simulink model "white_box"  (R2024b)
settings: Solver=ode1  StartTime=0.0  StopTime=Tobs  FixedStep=Ts  RelTol=1e-3
values from neighbouring files (symbols this model uses):
  delta_t = 10E-6    (= 1e-05)    [main_SVD.m]    (also in main_scan_FD.m)
  f0 = 50    [main_SVD.m]    (also in main_scan_FD.m)
  Id_ss = 0    [main_scan_FD.m]
  Ipeak = Sbase/Vpeak    [main_scan_FD.m]
  Iq_ss = 0    [main_scan_FD.m]
  P_finalvalue = 0.486    [main_scan_FD.m]    (also in main_ss_composite.m = 0.05)
  P_step_time = 1.5    [main_scan_FD.m]    (also in main_ss_composite.m = 10)
  phi = 0 * pi / 180    (= 0)    [main_SVD.m]
  signal_type = 1    [main_scan_FD.m]
  Ts = delta_t    (= 1e-05)    [main_scan_FD.m]
  V_finalvalue = 0.99    [main_ss_composite.m]
  V_step_time = 100    [main_scan_FD.m]    (also in main_ss_composite.m = 10)
  Vd_ss = 0    [main_scan_FD.m]
  Vpeak = (Vbase/sqrt(3))*sqrt(2)    [main_scan_FD.m]
  Vq_ss = 0    [main_scan_FD.m]
undefined symbols (not defined in the file or in its folder): C_dc, C_filt, dist_time, dist_value_0, dist_value_a, dist_value_b, dist_value_c, dist_value_d, dist_value_n, dist_value_p, dist_value_q, fd, I_charge, Iss_type, ki_inner_d_pu, ki_inner_q_pu, ki_outer_P_pu, ki_outer_V_pu, ki_pll, kp_inner_d_pu, kp_inner_q_pu, kp_outer_P_pu, kp_outer_V_pu, kp_pll, L, L_base, L_grid, L_vsc, omega_b, P_base, R_grid, R_vsc, Rsource, t_charge, V_base, V_dc, Vss_type
libraries: spsThreePhaseVIMeasurementLib x19, spsControlledVoltageSourceLib x18, spsControlledCurrentSourceLib x14, slpidlib x5, spsThreePhaseSeriesRLCBranchLib x5, spsabctodq0Lib x4, spsGroundLib x3, eeGeneralControl x2, spsdq0toabcLib x2, simulink x2, spsLeadLagFilterLib x1, spsParallelRLCBranchLib x1
(part 1 of 3)
settings Model: SimulationMode=accelerator  Creator=osro  LastModifiedBy=nicolae.darii
settings SolverCC: AlgebraicLoopSolver=TrustRegion
settings DebuggingCC: UnconnectedInputMsg=warning  UnconnectedOutputMsg=warning  UnconnectedLineMsg=warning
settings ModelReferenceCC: EnableRefExpFcnMdlSchedulingChecks=on
settings RTWCC: GPUComputeCapability=3.5

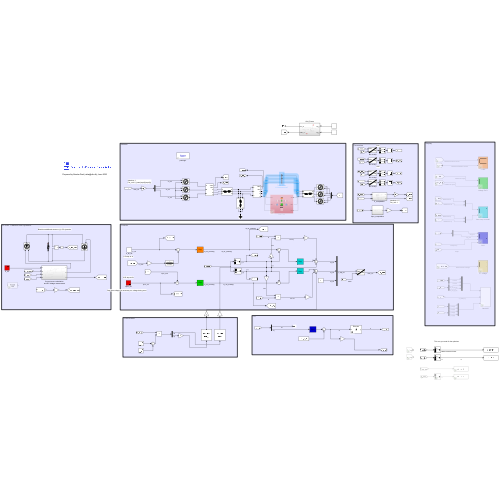
[thumbnail: Simulink's stored preview of the top-level diagram]
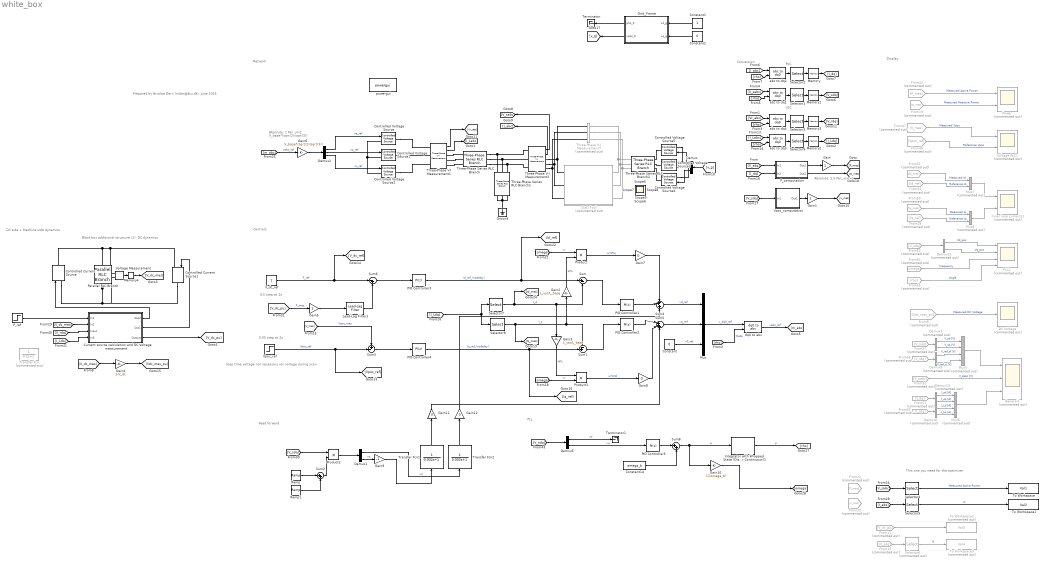
== system white_box ==
  note: Feed forward
  note: Step time voltage not necessary vor voltage during scan
  note: This one you need for the optimizer
  note: PLL
  note: 0.05 step at 2s
  note: 0.5 step at 1s
  note: Absolute: 1.5
      | Per_unit: 1
  note: Absolute: 1
      | Per_unit: V_base*(sqrt(2)/sqrt(3))
  note: Conversion
  note: Controls
  note: Network
  note: VSC
  note: PoC
  note: Prepared by Nicolae Darii (nidar@dtu.dk), June 2025
  note: DC side + Machine side dynamics
  note: Black box additional structure (1): DC dynamics
  note: Display
  Constant : Constant  Value=0
  Constant1 : Constant
  Constant14 : Constant  Value=omega_b
  Constant2 : Constant  Value=0
  Controlled Current Source : spsControlledCurrentSourceLib/Controlled Current Source  Initialize=on  Source_Type=AC  Amplitude=0  Phase=0  Frequency=0  Measurements=None
  Controlled Current Source1 : spsControlledCurrentSourceLib/Controlled Current Source  Initialize=on  Source_Type=AC  Amplitude=0  Phase=0  Frequency=0  Measurements=None
  Controlled Voltage Source{,1..5} (6 alike) : spsControlledVoltageSourceLib/Controlled Voltage Source  Initialize=on  Source_Type=AC  Amplitude=0  Phase=0  Frequency=0  Measurements=None
  Current source calculation and DC Voltage measurement : Subsystem
  DC Voltage : Scope  Commented=on
  Demux : Demux  Outputs=3
  Demux1 : Demux  Outputs=2
  Demux{7..11} (5 alike) : Demux  Commented=on  Outputs=2
  Demux2 : Demux  Outputs=3
  Demux5 : Demux  Outputs=2
  From11 : From  Commented=on  GotoTag=V_dc_pu
  From12 : From  Commented=on  GotoTag=V_sdq
  From19 : From  Commented=on  GotoTag=Q_mes
  From20 : From  Commented=on  GotoTag=V_mes
  From22 : From  Commented=on  GotoTag=P_mes
  From32 : From  Commented=on  GotoTag=V_sabc
  From35 : From  Commented=on  GotoTag=I_Ldq
  From37 : From  Commented=on  GotoTag=V_sdq
  From42 : From  Commented=on  GotoTag=P_mes
  From47 : From  Commented=on  GotoTag=V_mes
  From48 : From  Commented=on  GotoTag=Vpoc_ref
  From49 : From  Commented=on  GotoTag=Iq_ref
  From50 : From  Commented=on  GotoTag=Iq_mes
  From51 : From  Commented=on  GotoTag=Id_mes
  From52 : From  Commented=on  GotoTag=Id_ref
  From53 : From  Commented=on  GotoTag=V_sdq
  From54 : From  Commented=on  GotoTag=omega
  From55 : From  Commented=on  GotoTag=rho
  From56 : From  Commented=on  GotoTag=V_rdq
  From57 : From  Commented=on  GotoTag=I_dq
  From9 : From  Commented=on  GotoTag=Vdc_mes_pu
  Gain : Gain
  Gain1 : Gain
  Gain10 : Gain  Gain=1/(omega_b)
  Gain{7..8,11..12} (4 alike) : Gain  Gain=0
  Gain2 : Gain  Gain=L_vsc/L_base
  Gain3 : Gain  Gain=L_vsc/L_base
  Gain4 : Gain  Gain=1/V_dc
  Gain5 : Gain
  Gain6 : Gain  Gain=V_base*(sqrt(2)/sqrt(3))
  Gain9 : Gain  Gain=-1
  General1 : Scope  Commented=on  NumInputPorts=3
  Grid_Frame : Subsystem
  Ground : spsGroundLib/Ground  LConnTagsString=a
  Inner loop currents1 : Scope  Commented=on  NumInputPorts=2
  Integrator with Wrapped State (Discrete or Continuous)1 : eeGeneralControl/Integrator with Wrapped State (Discrete or Continuous)  LabelModeActiveChoice=Discrete  WrappedStateUpperValue=2*pi  WrappedStateLowerValue=0  x0=0  Ts=-1
  Lead-Lag Filter1 : spsLeadLagFilterLib/Lead-Lag Filter  T1=T1  T2=T2  Vdc_Init=1  Ts=Ts
      settings: LibrarySourceBlock=|
      | sps_lib/Control/Filters/Lead-Lag
      | Filter
  Memory{,1..3} (4 alike) : Memory  InitialCondition=[0 0]  InheritSampleTime=on  LinearizeMemory=on  LinearizeAsDelay=on
  Memory4 : Memory
  Mux : Mux  Inputs=3
  Mux5 : Mux  Commented=on
  Mux6 : Mux  Commented=on
  Mux7 : Mux  Commented=on  Inputs=2
  Mux8 : Mux  Commented=on  Inputs=2
  PID Controller1 : slpidlib/PID Controller  Controller=PI  Form=Parallel  TimeDomain=Discrete-time  UseExternalTs=off  SampleTime=Ts  IntegratorMethod=Forward Euler  FilterMethod=Forward Euler  ControllerParametersSource=internal  P=kp_inner_d_pu  I=ki_inner_d_pu  UseKiTs=off  D=0  UseExternalDerivativeSource=off  N=100  UseFilter=on  TunerSelectOption=Transfer Function Based (PID Tuner App)  InitialConditionSource=internal  InitialConditionForIntegrator=0  InitialConditionForFilter=0  DifferentiatorICPrevScaledInput=0  ExternalReset=none  TrackingMode=off  Kt=1  LimitOutput=off  SatLimitsSource=internal  UpperSaturationLimit=inf  LowerSaturationLimit=-inf  LinearizeAsGain=on  AntiWindupMode=none  Kb=1  LimitIntegrator=off  UpperIntegratorSaturationLimit=inf  LowerIntegratorSaturationLimit=-inf  POutMin=[]  POutMax=[]  IOutMin=[]  IOutMax=[]  DOutMin=[]  DOutMax=[]  NOutMin=[]  NOutMax=[]  SumOutMin=[]  SumOutMax=[]  SaturationOutMin=[]  SaturationOutMax=[]  PParamMin=[]  PParamMax=[]  IParamMin=[]  IParamMax=[]  DParamMin=[]  DParamMax=[]  NParamMin=[]  NParamMax=[]  KbParamMin=[]  KbParamMax=[]  KtParamMin=[]  KtParamMax=[]  KbOutMin=[]  KbOutMax=[]  KtOutMin=[]  KtOutMax=[]  IntegratorOutMin=[]  IntegratorOutMax=[]  FilterOutMin=[]  FilterOutMax=[]  SumI1OutMin=[]  SumI1OutMax=[]  SumI2OutMin=[]  SumI2OutMax=[]  SumI3OutMin=[]  SumI3OutMax=[]  SumI4OutMin=[]  SumI4OutMax=[]  SumDOutMin=[]  SumDOutMax=[]  DifferentiatorOutMin=[]  DifferentiatorOutMax=[]  FilterDiffOutCoefMin=[]  FilterDiffOutCoefMax=[]  ReciprocalOutMin=[]  ReciprocalOutMax=[]  SumDenOutMin=[]  SumDenOutMax=[]  SumNumOutMin=[]  SumNumOutMax=[]  DivideOutMin=[]  DivideOutMax=[]  UdiffTsProdOutMin=[]  UdiffTsProdOutMax=[]  NTsProdOutMin=[]  NTsProdOutMax=[]  UintegralTsProdOutMin=[]  UintegralTsProdOutMax=[]  UngainTsProdOutMin=[]  UngainTsProdOutMax=[]  ClampingZeroOutDataTypeStr=Inherit: Inherit via back propagation  ClampingZeroOutMin=[]  ClampingZeroOutMax=[]  FilterDenConstantOutDataTypeStr=Inherit: Inherit via back propagation  FilterDenConstantOutMin=[]  FilterDenConstantOutMax=[]  PCopyOutDataTypeStr=Inherit: Inherit via back propagation  PCopyOutMin=[]  PCopyOutMax=[]  NCopyOutDataTypeStr=Inherit: Inherit via back propagation  NCopyOutMin=[]  NCopyOutMax=[]  IntegratorContinuousStateAttributes=''  IntegratorStateMustResolveToSignalObject=off  IntegratorRTWStateStorageClass=Auto  FilterContinuousStateAttributes=''  FilterStateMustResolveToSignalObject=off  FilterRTWStateStorageClass=Auto  ParallelPVariant=InternalParameters  IdealPVariant=Disabled  IVariant=InternalParameters  DVariant=Disabled  IntegratorVariant=Discrete  SatVariant=Disabled  AWVariant=Passthrough  PCopyVariant=Disabled  TRVariant=Disabled  FdbkBlocksVariant=Forward  IdealPFdbkVariant=Disabled  SatFdbkVariant=Disabled  DerivativeFilterVariant=Disabled  NVariant=Disabled  NCopyVariant=Disabled_SignalSpec  FilterICVariant=Disabled  IntegratorICVariant=InternalICs  ExternalResetVariant=Disabled  TRSumVariant=Passthrough  SumFdbkVariant=Disabled  SumVariant=Sum_PI  TsampFilterVariant=InternalTs  TsampNgainVariant=Passthrough  TsampIntegralVariant=Disabled_SignalSpec  ExternalSaturationOutDataTypeStr=Inherit: Same as second input  DerivativeSourceVariant=Disabled  PreIntVariant=InternalPreInt
  PID Controller2 : slpidlib/PID Controller  Controller=PI  Form=Parallel  TimeDomain=Discrete-time  UseExternalTs=off  SampleTime=Ts  IntegratorMethod=Forward Euler  FilterMethod=Forward Euler  ControllerParametersSource=internal  P=kp_inner_q_pu  I=ki_inner_q_pu  UseKiTs=off  D=0  UseExternalDerivativeSource=off  N=100  UseFilter=on  TunerSelectOption=Transfer Function Based (PID Tuner App)  InitialConditionSource=internal  InitialConditionForIntegrator=0  InitialConditionForFilter=0  DifferentiatorICPrevScaledInput=0  ExternalReset=none  TrackingMode=off  Kt=1  LimitOutput=off  SatLimitsSource=internal  UpperSaturationLimit=inf  LowerSaturationLimit=-inf  LinearizeAsGain=on  AntiWindupMode=none  Kb=1  LimitIntegrator=off  UpperIntegratorSaturationLimit=inf  LowerIntegratorSaturationLimit=-inf  POutMin=[]  POutMax=[]  IOutMin=[]  IOutMax=[]  DOutMin=[]  DOutMax=[]  NOutMin=[]  NOutMax=[]  SumOutMin=[]  SumOutMax=[]  SaturationOutMin=[]  SaturationOutMax=[]  PParamMin=[]  PParamMax=[]  IParamMin=[]  IParamMax=[]  DParamMin=[]  DParamMax=[]  NParamMin=[]  NParamMax=[]  KbParamMin=[]  KbParamMax=[]  KtParamMin=[]  KtParamMax=[]  KbOutMin=[]  KbOutMax=[]  KtOutMin=[]  KtOutMax=[]  IntegratorOutMin=[]  IntegratorOutMax=[]  FilterOutMin=[]  FilterOutMax=[]  SumI1OutMin=[]  SumI1OutMax=[]  SumI2OutMin=[]  SumI2OutMax=[]  SumI3OutMin=[]  SumI3OutMax=[]  SumI4OutMin=[]  SumI4OutMax=[]  SumDOutMin=[]  SumDOutMax=[]  DifferentiatorOutMin=[]  DifferentiatorOutMax=[]  FilterDiffOutCoefMin=[]  FilterDiffOutCoefMax=[]  ReciprocalOutMin=[]  ReciprocalOutMax=[]  SumDenOutMin=[]  SumDenOutMax=[]  SumNumOutMin=[]  SumNumOutMax=[]  DivideOutMin=[]  DivideOutMax=[]  UdiffTsProdOutMin=[]  UdiffTsProdOutMax=[]  NTsProdOutMin=[]  NTsProdOutMax=[]  UintegralTsProdOutMin=[]  UintegralTsProdOutMax=[]  UngainTsProdOutMin=[]  UngainTsProdOutMax=[]  ClampingZeroOutDataTypeStr=Inherit: Inherit via back propagation  ClampingZeroOutMin=[]  ClampingZeroOutMax=[]  FilterDenConstantOutDataTypeStr=Inherit: Inherit via back propagation  FilterDenConstantOutMin=[]  FilterDenConstantOutMax=[]  PCopyOutDataTypeStr=Inherit: Inherit via back propagation  PCopyOutMin=[]  PCopyOutMax=[]  NCopyOutDataTypeStr=Inherit: Inherit via back propagation  NCopyOutMin=[]  NCopyOutMax=[]  IntegratorContinuousStateAttributes=''  IntegratorStateMustResolveToSignalObject=off  IntegratorRTWStateStorageClass=Auto  FilterContinuousStateAttributes=''  FilterStateMustResolveToSignalObject=off  FilterRTWStateStorageClass=Auto  ParallelPVariant=InternalParameters  IdealPVariant=Disabled  IVariant=InternalParameters  DVariant=Disabled  IntegratorVariant=Discrete  SatVariant=Disabled  AWVariant=Passthrough  PCopyVariant=Disabled  TRVariant=Disabled  FdbkBlocksVariant=Forward  IdealPFdbkVariant=Disabled  SatFdbkVariant=Disabled  DerivativeFilterVariant=Disabled  NVariant=Disabled  NCopyVariant=Disabled_SignalSpec  FilterICVariant=Disabled  IntegratorICVariant=InternalICs  ExternalResetVariant=Disabled  TRSumVariant=Passthrough  SumFdbkVariant=Disabled  SumVariant=Sum_PI  TsampFilterVariant=InternalTs  TsampNgainVariant=Passthrough  TsampIntegralVariant=Disabled_SignalSpec  ExternalSaturationOutDataTypeStr=Inherit: Same as second input  DerivativeSourceVariant=Disabled  PreIntVariant=InternalPreInt
  PID Controller3 : slpidlib/PID Controller  Controller=PI  Form=Parallel  TimeDomain=Discrete-time  UseExternalTs=off  SampleTime=Ts  IntegratorMethod=Forward Euler  FilterMethod=Forward Euler  ControllerParametersSource=internal  P=kp_outer_P_pu  I=ki_outer_P_pu  UseKiTs=off  D=0  UseExternalDerivativeSource=off  N=100  UseFilter=on  TunerSelectOption=Transfer Function Based (PID Tuner App)  InitialConditionSource=internal  InitialConditionForIntegrator=0  InitialConditionForFilter=0  DifferentiatorICPrevScaledInput=0  ExternalReset=none  TrackingMode=off  Kt=1  LimitOutput=off  SatLimitsSource=internal  UpperSaturationLimit=inf  LowerSaturationLimit=-inf  LinearizeAsGain=on  AntiWindupMode=none  Kb=1  LimitIntegrator=off  UpperIntegratorSaturationLimit=inf  LowerIntegratorSaturationLimit=-inf  POutMin=[]  POutMax=[]  IOutMin=[]  IOutMax=[]  DOutMin=[]  DOutMax=[]  NOutMin=[]  NOutMax=[]  SumOutMin=[]  SumOutMax=[]  SaturationOutMin=[]  SaturationOutMax=[]  PParamMin=[]  PParamMax=[]  IParamMin=[]  IParamMax=[]  DParamMin=[]  DParamMax=[]  NParamMin=[]  NParamMax=[]  KbParamMin=[]  KbParamMax=[]  KtParamMin=[]  KtParamMax=[]  KbOutMin=[]  KbOutMax=[]  KtOutMin=[]  KtOutMax=[]  IntegratorOutMin=[]  IntegratorOutMax=[]  FilterOutMin=[]  FilterOutMax=[]  SumI1OutMin=[]  SumI1OutMax=[]  SumI2OutMin=[]  SumI2OutMax=[]  SumI3OutMin=[]  SumI3OutMax=[]  SumI4OutMin=[]  SumI4OutMax=[]  SumDOutMin=[]  SumDOutMax=[]  DifferentiatorOutMin=[]  DifferentiatorOutMax=[]  FilterDiffOutCoefMin=[]  FilterDiffOutCoefMax=[]  ReciprocalOutMin=[]  ReciprocalOutMax=[]  SumDenOutMin=[]  SumDenOutMax=[]  SumNumOutMin=[]  SumNumOutMax=[]  DivideOutMin=[]  DivideOutMax=[]  UdiffTsProdOutMin=[]  UdiffTsProdOutMax=[]  NTsProdOutMin=[]  NTsProdOutMax=[]  UintegralTsProdOutMin=[]  UintegralTsProdOutMax=[]  UngainTsProdOutMin=[]  UngainTsProdOutMax=[]  ClampingZeroOutDataTypeStr=Inherit: Inherit via back propagation  ClampingZeroOutMin=[]  ClampingZeroOutMax=[]  FilterDenConstantOutDataTypeStr=Inherit: Inherit via back propagation  FilterDenConstantOutMin=[]  FilterDenConstantOutMax=[]  PCopyOutDataTypeStr=Inherit: Inherit via back propagation  PCopyOutMin=[]  PCopyOutMax=[]  NCopyOutDataTypeStr=Inherit: Inherit via back propagation  NCopyOutMin=[]  NCopyOutMax=[]  IntegratorContinuousStateAttributes=''  IntegratorStateMustResolveToSignalObject=off  IntegratorRTWStateStorageClass=Auto  FilterContinuousStateAttributes=''  FilterStateMustResolveToSignalObject=off  FilterRTWStateStorageClass=Auto  ParallelPVariant=InternalParameters  IdealPVariant=Disabled  IVariant=InternalParameters  DVariant=Disabled  IntegratorVariant=Discrete  SatVariant=Disabled  AWVariant=Passthrough  PCopyVariant=Disabled  TRVariant=Disabled  FdbkBlocksVariant=Forward  IdealPFdbkVariant=Disabled  SatFdbkVariant=Disabled  DerivativeFilterVariant=Disabled  NVariant=Disabled  NCopyVariant=Disabled_SignalSpec  FilterICVariant=Disabled  IntegratorICVariant=InternalICs  ExternalResetVariant=Disabled  TRSumVariant=Passthrough  SumFdbkVariant=Disabled  SumVariant=Sum_PI  TsampFilterVariant=InternalTs  TsampNgainVariant=Passthrough  TsampIntegralVariant=Disabled_SignalSpec  ExternalSaturationOutDataTypeStr=Inherit: Same as second input  DerivativeSourceVariant=Disabled  PreIntVariant=InternalPreInt
  PID Controller4 : slpidlib/PID Controller  Controller=PI  Form=Parallel  TimeDomain=Discrete-time  UseExternalTs=off  SampleTime=Ts  IntegratorMethod=Forward Euler  FilterMethod=Forward Euler  ControllerParametersSource=internal  P=abs(kp_outer_V_pu)  I=abs(ki_outer_V_pu)  UseKiTs=off  D=0  UseExternalDerivativeSource=off  N=100  UseFilter=on  TunerSelectOption=Transfer Function Based (PID Tuner App)  InitialConditionSource=internal  InitialConditionForIntegrator=0  InitialConditionForFilter=0  DifferentiatorICPrevScaledInput=0  ExternalReset=none  TrackingMode=off  Kt=1  LimitOutput=off  SatLimitsSource=internal  UpperSaturationLimit=inf  LowerSaturationLimit=-inf  LinearizeAsGain=on  AntiWindupMode=none  Kb=1  LimitIntegrator=off  UpperIntegratorSaturationLimit=inf  LowerIntegratorSaturationLimit=-inf  POutMin=[]  POutMax=[]  IOutMin=[]  IOutMax=[]  DOutMin=[]  DOutMax=[]  NOutMin=[]  NOutMax=[]  SumOutMin=[]  SumOutMax=[]  SaturationOutMin=[]  SaturationOutMax=[]  PParamMin=[]  PParamMax=[]  IParamMin=[]  IParamMax=[]  DParamMin=[]  DParamMax=[]  NParamMin=[]  NParamMax=[]  KbParamMin=[]  KbParamMax=[]  KtParamMin=[]  KtParamMax=[]  KbOutMin=[]  KbOutMax=[]  KtOutMin=[]  KtOutMax=[]  IntegratorOutMin=[]  IntegratorOutMax=[]  FilterOutMin=[]  FilterOutMax=[]  SumI1OutMin=[]  SumI1OutMax=[]  SumI2OutMin=[]  SumI2OutMax=[]  SumI3OutMin=[]  SumI3OutMax=[]  SumI4OutMin=[]  SumI4OutMax=[]  SumDOutMin=[]  SumDOutMax=[]  DifferentiatorOutMin=[]  DifferentiatorOutMax=[]  FilterDiffOutCoefMin=[]  FilterDiffOutCoefMax=[]  ReciprocalOutMin=[]  ReciprocalOutMax=[]  SumDenOutMin=[]  SumDenOutMax=[]  SumNumOutMin=[]  SumNumOutMax=[]  DivideOutMin=[]  DivideOutMax=[]  UdiffTsProdOutMin=[]  UdiffTsProdOutMax=[]  NTsProdOutMin=[]  NTsProdOutMax=[]  UintegralTsProdOutMin=[]  UintegralTsProdOutMax=[]  UngainTsProdOutMin=[]  UngainTsProdOutMax=[]  ClampingZeroOutDataTypeStr=Inherit: Inherit via back propagation  ClampingZeroOutMin=[]  ClampingZeroOutMax=[]  FilterDenConstantOutDataTypeStr=Inherit: Inherit via back propagation  FilterDenConstantOutMin=[]  FilterDenConstantOutMax=[]  PCopyOutDataTypeStr=Inherit: Inherit via back propagation  PCopyOutMin=[]  PCopyOutMax=[]  NCopyOutDataTypeStr=Inherit: Inherit via back propagation  NCopyOutMin=[]  NCopyOutMax=[]  IntegratorContinuousStateAttributes=''  IntegratorStateMustResolveToSignalObject=off  IntegratorRTWStateStorageClass=Auto  FilterContinuousStateAttributes=''  FilterStateMustResolveToSignalObject=off  FilterRTWStateStorageClass=Auto  ParallelPVariant=InternalParameters  IdealPVariant=Disabled  IVariant=InternalParameters  DVariant=Disabled  IntegratorVariant=Discrete  SatVariant=Disabled  AWVariant=Passthrough  PCopyVariant=Disabled  TRVariant=Disabled  FdbkBlocksVariant=Forward  IdealPFdbkVariant=Disabled  SatFdbkVariant=Disabled  DerivativeFilterVariant=Disabled  NVariant=Disabled  NCopyVariant=Disabled_SignalSpec  FilterICVariant=Disabled  IntegratorICVariant=InternalICs  ExternalResetVariant=Disabled  TRSumVariant=Passthrough  SumFdbkVariant=Disabled  SumVariant=Sum_PI  TsampFilterVariant=InternalTs  TsampNgainVariant=Passthrough  TsampIntegralVariant=Disabled_SignalSpec  ExternalSaturationOutDataTypeStr=Inherit: Same as second input  DerivativeSourceVariant=Disabled  PreIntVariant=InternalPreInt
  PID Controller5 : slpidlib/PID Controller  Controller=PI  Form=Parallel  TimeDomain=Discrete-time  UseExternalTs=off  SampleTime=Ts  IntegratorMethod=Forward Euler  FilterMethod=Forward Euler  ControllerParametersSource=internal  P=kp_pll  I=ki_pll  UseKiTs=off  D=0  UseExternalDerivativeSource=off  N=100  UseFilter=on  TunerSelectOption=Transfer Function Based (PID Tuner App)  InitialConditionSource=internal  InitialConditionForIntegrator=0  InitialConditionForFilter=0  DifferentiatorICPrevScaledInput=0  ExternalReset=none  TrackingMode=off  Kt=1  LimitOutput=off  SatLimitsSource=internal  UpperSaturationLimit=inf  LowerSaturationLimit=-inf  LinearizeAsGain=on  AntiWindupMode=none  Kb=1  LimitIntegrator=off  UpperIntegratorSaturationLimit=inf  LowerIntegratorSaturationLimit=-inf  POutMin=[]  POutMax=[]  IOutMin=[]  IOutMax=[]  DOutMin=[]  DOutMax=[]  NOutMin=[]  NOutMax=[]  SumOutMin=[]  SumOutMax=[]  SaturationOutMin=[]  SaturationOutMax=[]  PParamMin=[]  PParamMax=[]  IParamMin=[]  IParamMax=[]  DParamMin=[]  DParamMax=[]  NParamMin=[]  NParamMax=[]  KbParamMin=[]  KbParamMax=[]  KtParamMin=[]  KtParamMax=[]  KbOutMin=[]  KbOutMax=[]  KtOutMin=[]  KtOutMax=[]  IntegratorOutMin=[]  IntegratorOutMax=[]  FilterOutMin=[]  FilterOutMax=[]  SumI1OutMin=[]  SumI1OutMax=[]  SumI2OutMin=[]  SumI2OutMax=[]  SumI3OutMin=[]  SumI3OutMax=[]  SumI4OutMin=[]  SumI4OutMax=[]  SumDOutMin=[]  SumDOutMax=[]  DifferentiatorOutMin=[]  DifferentiatorOutMax=[]  FilterDiffOutCoefMin=[]  FilterDiffOutCoefMax=[]  ReciprocalOutMin=[]  ReciprocalOutMax=[]  SumDenOutMin=[]  SumDenOutMax=[]  SumNumOutMin=[]  SumNumOutMax=[]  DivideOutMin=[]  DivideOutMax=[]  UdiffTsProdOutMin=[]  UdiffTsProdOutMax=[]  NTsProdOutMin=[]  NTsProdOutMax=[]  UintegralTsProdOutMin=[]  UintegralTsProdOutMax=[]  UngainTsProdOutMin=[]  UngainTsProdOutMax=[]  ClampingZeroOutDataTypeStr=Inherit: Inherit via back propagation  ClampingZeroOutMin=[]  ClampingZeroOutMax=[]  FilterDenConstantOutDataTypeStr=Inherit: Inherit via back propagation  FilterDenConstantOutMin=[]  FilterDenConstantOutMax=[]  PCopyOutDataTypeStr=Inherit: Inherit via back propagation  PCopyOutMin=[]  PCopyOutMax=[]  NCopyOutDataTypeStr=Inherit: Inherit via back propagation  NCopyOutMin=[]  NCopyOutMax=[]  IntegratorContinuousStateAttributes=''  IntegratorStateMustResolveToSignalObject=off  IntegratorRTWStateStorageClass=Auto  FilterContinuousStateAttributes=''  FilterStateMustResolveToSignalObject=off  FilterRTWStateStorageClass=Auto  ParallelPVariant=InternalParameters  IdealPVariant=Disabled  IVariant=InternalParameters  DVariant=Disabled  IntegratorVariant=Discrete  SatVariant=Disabled  AWVariant=Passthrough  PCopyVariant=Disabled  TRVariant=Disabled  FdbkBlocksVariant=Forward  IdealPFdbkVariant=Disabled  SatFdbkVariant=Disabled  DerivativeFilterVariant=Disabled  NVariant=Disabled  NCopyVariant=Disabled_SignalSpec  FilterICVariant=Disabled  IntegratorICVariant=InternalICs  ExternalResetVariant=Disabled  TRSumVariant=Passthrough  SumFdbkVariant=Disabled  SumVariant=Sum_PI  TsampFilterVariant=InternalTs  TsampNgainVariant=Passthrough  TsampIntegralVariant=Disabled_SignalSpec  ExternalSaturationOutDataTypeStr=Inherit: Same as second input  DerivativeSourceVariant=Disabled  PreIntVariant=InternalPreInt
  PLL1 : Scope  Commented=on  NumInputPorts=4
  P_computation : Subsystem
  P_ref : Step  Time=P_step_time  After=P_finalvalue  SampleTime=0
  Parallel RLC Branch : spsParallelRLCBranchLib/Parallel RLC Branch  LConnTagsString=a  RConnTagsString=__new0  BranchType=C  Resistance=1  Inductance=1e-3  SetiL0=off  InitialCurrent=0  Capacitance=C_dc  Setx0=on  InitialVoltage=0  Measurements=None
  Power : Scope  Commented=on  NumInputPorts=2
  Product : Product
  Product1 : Product
  Product2 : Product
  Ramp : simulink/Sources/Ramp  slope=1  start=0  InitialOutput=0
  Ramp1 : simulink/Sources/Ramp  slope=-1  start=1  InitialOutput=0
  SIaD Tool : Subsystem  Commented=on
  Selector{1..3,9} (4 alike) : Selector  InputPortWidth=3  IndexOptions=Index vector (dialog)  Indices=[1 2]  OutputSizes=1
  Selector4 : Selector  InputPortWidth=3  IndexOptions=Index vector (dialog)  Indices=[1]  OutputSizes=1
  Selector5 : Selector  InputPortWidth=3  IndexOptions=Index vector (dialog)  Indices=[1]  OutputSizes=1
  Selector6 : Selector  Commented=on  InputPortWidth=2  IndexOptions=Index vector (dialog)  Indices=[2]  OutputSizes=1
  Selector7 : Selector  InputPortWidth=2  IndexOptions=Index vector (dialog)  Indices=[1]  OutputSizes=1
  Selector8 : Selector  InputPortWidth=2  IndexOptions=Index vector (dialog)  Indices=[2]  OutputSizes=1
  Sum : Sum  Inputs=|+-
  Sum1 : Sum  Inputs=-+|
  Sum2 : Sum  Inputs=|++
  Sum3 : Sum  Inputs=+-|
  Sum4 : Sum  Inputs=-+|+
  Sum5 : Sum  Inputs=|+++
  Sum6 : Sum  Inputs=|-+
  Sum8 : Sum  Inputs=|++
  Terminator : Terminator
  Terminator1 : Terminator
  Three-Phase Series RLC Branch : spsThreePhaseSeriesRLCBranchLib/Three-Phase Series RLC Branch  LConnTagsString=A|B|C  RConnTagsString=A|B|C  BranchType=RL  Resistance=R_vsc  Inductance=L_vsc  Capacitance=1e-6  Measurements=None
  Three-Phase Series RLC Branch1 : spsThreePhaseSeriesRLCBranchLib/Three-Phase Series RLC Branch  LConnTagsString=A|B|C  RConnTagsString=A|B|C  BranchType=RC  Resistance=0  Inductance=L  Capacitance=C_filt  Measurements=None
  Three-Phase Series RLC Branch2 : spsThreePhaseSeriesRLCBranchLib/Three-Phase Series RLC Branch  LConnTagsString=A|B|C  RConnTagsString=A|B|C  BranchType=RL  Resistance=R_grid  Inductance=L_grid  Capacitance=1e-6  Measurements=None
  Three-Phase V-I Measurement1 : spsThreePhaseVIMeasurementLib/Three-Phase V-I Measurement  VoltageMeasurement=phase-to-ground  SetLabelV=off  LabelV=Vabc  Vpu=on  VpuLL=off  CurrentMeasurement=yes  SetLabelI=off  LabelI=Iabc  Ipu=on  Pbase=P_base  Vbase=V_base  OutputType=Complex  PhasorSimulation=off  PSBequivalent=0
  Three-Phase V-I Measurement2 : spsThreePhaseVIMeasurementLib/Three-Phase V-I Measurement  VoltageMeasurement=phase-to-ground  SetLabelV=off  LabelV=Vabc  Vpu=on  VpuLL=off  CurrentMeasurement=yes  SetLabelI=off  LabelI=Iabc  Ipu=on  Pbase=P_base  Vbase=V_base  OutputType=Complex  PhasorSimulation=off  PSBequivalent=0
  Three-Phase V-I Measurement7 : spsThreePhaseVIMeasurementLib/Three-Phase V-I Measurement  Commented=on  VoltageMeasurement=no  SetLabelV=on  LabelV=Vabc  Vpu=off  VpuLL=off  CurrentMeasurement=no  SetLabelI=on  LabelI=Iabc  Ipu=off  Pbase=100e6  Vbase=500e3  OutputType=Complex  PhasorSimulation=off  PSBequivalent=0
  To Workspace : ToWorkspace  VariableName=Val1  SaveFormat=Structure With Time  SampleTime=-1
  To Workspace1 : ToWorkspace  VariableName=Val2  SaveFormat=Structure With Time  SampleTime=-1
  To Workspace2 : ToWorkspace  Commented=on  VariableName=Val3  SaveFormat=Structure With Time  SampleTime=-1
  To Workspace3 : ToWorkspace  Commented=on  VariableName=Val4  SaveFormat=Structure With Time  SampleTime=-1
  Transfer Fcn : TransferFcn  Commented=on  Denominator=[0.2 1]
  Transfer Fcn1 : TransferFcn  Denominator=[0.002 1]
  Transfer Fcn2 : TransferFcn  Denominator=[0.002 1]
  V_dc_ref : Constant
  Voltage Measurement : spsVoltageMeasurementLib/Voltage Measurement  PhasorSimulation=off  OutputType=Complex  PSBequivalent=0
  Voltage PoC1 : Scope  Commented=on  NumInputPorts=2
  Vpoc_computation : Subsystem
  Vpoc_ref : Step  Time=V_step_time  Before=1  After=V_finalvalue  SampleTime=0
  abc to dq{1..4} (4 alike) : spsabctodq0Lib/abc to dq0  Alignment=90 degrees behind phase A axis
  dq0 to abc : spsdq0toabcLib/dq0 to abc  Alignment=90 degrees behind phase A axis
  powergui : sps_lib/powergui  Priority=1  SimulationMode=Discrete  SampleTime=Ts  frequency=60  Iterations=50  frequencyindice=0  Pbase=100e6  ErrMax=1e-4  UnitsV=kV  UnitsW=MW  buscounter=0  FunctionMessages=on  echomessages=off  EnableUseOfTLC=off  CurrentSourceSwitches=off  DisableSnubberDevices=off  DisableRonSwitches=off  DisableVfSwitches=off  DisplayEquations=off  AutomaticDiscreteSolvers=off  SolverType=Tustin/Backward Euler (TBE)  Interpol=off  ExternalGateDelay=off  methode=off  Ts=100  x0status=zero  SPID=on  SwTol=0  HookPort=off  NonlinearTolerance=1e-4  nMaxIteration=100  ContinueOnMaxIteration=off  RestoreLinks=warning  ResistiveCurrentMeasurement=off  Frange=[0:2:500]  Ylog=off  Xlog=on  ShowGrid=off  save=off  variable=ZData  structure=0  ZoomFFT=off  StartTime=0.0  cycles=1  DisplayStyle=1  fundamental=60  FreqAxis=off  MaxFrequency=1000  frequencyindicesteady=1  RmsSteady=1  display=off
  Scope{2,5..9} (6 alike) : Scope
  wires:
  Selector1/1 -> Memory1/1
  abc to dq1/1 -> Selector1/1
  [rho] -> dq0 to abc/2  "theta"
  [V_sabc] -> abc to dq1/1
  [rho] -> abc to dq1/2
  [rho] -> abc to dq2/2
  Selector2/1 -> Memory/1
  [I_abc] -> abc to dq2/1
  abc to dq2/1 -> Selector2/1
  Constant/1 -> Mux/3  "v0_ref"
  Three-Phase V-I Measurement1/2 -> [I_Labc]
  Memory/1 -> [I_dq]
  Memory1/1 -> [V_sdq]
  Three-Phase V-I Measurement2/1 -> [V_sabc]
  Three-Phase V-I Measurement2/2 -> [I_abc]
  Memory2/1 -> [I_Ldq]
  abc to dq3/1 -> Selector9/1
  [I_Labc] -> abc to dq3/1
  Selector9/1 -> Memory2/1
  [rho] -> abc to dq3/2
  [V_sdq] -> P_computation/1(In1)
  [I_dq] -> P_computation/2(In2)
  P_computation/1(Out1) -> Gain/1
  [V_sdq] -> Vpoc_computation/1(In1)
  Vpoc_computation/1(Out1) -> Gain1/1
  Gain6/1 -> Demux2/1
  Demux2/1 -> Controlled Voltage Source/1  "va_ref"
  Demux2/2 -> Controlled Voltage Source1/1  "vb_ref"
  Demux2/3 -> Controlled Voltage Source2/1  "vc_ref"
  Three-Phase V-I Measurement1/1 -> [Vr_abc]
  [m_abc] -> Gain6/1  "vabc_ref"
  Selector7/1 -> Gain3/1, Sum/2, [Id_mes]  "I_d"
  [I_Ldq] -> Selector8/1, Selector7/1
  Selector8/1 -> Gain2/1, Sum1/1, [Iq_mes]  "I_q"
  Sum/1 -> PID Controller1/1
  Sum1/1 -> PID Controller2/1
  [rho] -> abc to dq4/2
  Selector3/1 -> Memory3/1
  Memory3/1 -> [V_rdq]
  abc to dq4/1 -> Selector3/1
  [Vr_abc] -> abc to dq4/1
  [V_mes] -> Sum3/1  "Vpoc_mes"
  Vpoc_ref/1 -> [Vpoc_ref], Sum3/2  "Vpoc_ref"
  dq0 to abc/1 -> [m_abc]  "vabc_ref"
  Gain/1 -> [P_mes]
  Gain1/1 -> [V_mes]
  PID Controller4/1 -> [Iq_ref], Sum1/2  "Iq_ref_(nodelay)"
  [omega] -> Product/1  "w"
  Gain2/1 -> Product/2  "Iq*L"
  [omega] -> Product1/2  "w"
  Gain3/1 -> Product1/1  "Id*L"
  PID Controller1/1 -> Sum4/2
  Sum4/1 -> Mux/1  "vd_ref"
  Product/1 -> Gain7/1  "w*L*Iq"
  PID Controller2/1 -> Sum5/1
  Sum5/1 -> Mux/2  "vq_ref"
  Product1/1 -> Gain8/1  "w*L*Id"
  PID Controller3/1 -> [Id_ref], Sum/1  "Id_ref_(nodelay)"
  Demux5/1 -> Terminator1/1  "vd"
  [V_sdq] -> Demux5/1
  Constant14/1 -> Sum8/2
  Sum8/1 -> Gain10/1, Integrator with Wrapped State (Discrete or Continuous)1/1  "w"
  PID Controller5/1 -> Sum8/1
  Integrator with Wrapped State (Discrete or Continuous)1/1 -> [rho]  "p"
  Mux/1 -> dq0 to abc/1  "v_dq0_ref"
  Gain10/1 -> [omega]
  Selector5/1 -> To Workspace1/1  "I1"
  [V_sabc] -> Selector4/1
  [I_abc] -> Selector5/1
  [V_rdq] -> Current source calculation and DC Voltage measurement/3(Input)
  Voltage Measurement/1 -> Memory4/1
  Current source calculation and DC Voltage measurement/1(Out2) -> Controlled Current Source/1
  [I_Ldq] -> Current source calculation and DC Voltage measurement/4(In3)
  Current source calculation and DC Voltage measurement/2(Out1) -> Controlled Current Source1/1
  Memory4/1 -> [V_dc_mes]
  Current source calculation and DC Voltage measurement/3(Output) -> [V_dc_pu]
  [V_dc_mes] -> Current source calculation and DC Voltage measurement/2(In2)
  Sum6/1 -> PID Controller3/1
  V_dc_ref/1 -> [V_dc_ref], Sum6/1  "P_ref"
  Demux9/2 -> Mux5/4  "V_ref_q [V]"
  From9/1 -> DC Voltage/1  "Measured DC Voltage"
  From55/1 -> PLL1/4  "Angle"
  From35/1 -> Demux8/1
  From57/1 -> Demux10/1
  From54/1 -> PLL1/3  "Frequency"
  From47/1 -> Voltage PoC1/1  "Measured Vpoc"
  Demux11/2 -> PLL1/2  "Vq_poc"
  Demux8/2 -> Mux6/4  "I_Lq [A]"
  From50/1 -> Mux8/1  "Measured Iq"
  Demux10/1 -> Mux6/1  "I_sd [A]"
  Mux6/1 -> General1/3
  Demux11/1 -> PLL1/1  "Vd_poc"
  Demux7/2 -> Mux5/2  "V_sq [V]"
  From51/1 -> Mux7/1  "Measured Id"
  From56/1 -> Demux9/1
  Demux8/1 -> Mux6/3  "I_Ld [A]"
  From48/1 -> Voltage PoC1/2  "Reference Vpoc"
  From53/1 -> Demux11/1
  From49/1 -> Mux8/2  "Reference Iq"
  Mux8/1 -> Inner loop currents1/2
  From42/1 -> Power/1  "Measured Active Power"
  Mux5/1 -> General1/1
  From32/1 -> General1/2  "V_sabc [V]"
  Demux10/2 -> Mux6/2  "I_sq [A]"
  Demux7/1 -> Mux5/1  "V_sd [V]"
  Demux9/1 -> Mux5/3  "V_ref_d [V]"
  From52/1 -> Mux7/2  "Reference Id"
  Mux7/1 -> Inner loop currents1/1
  From37/1 -> Demux7/1
  [V_dc_mes] -> Gain4/1
  Gain4/1 -> [Vdc_mes_pu]
  From11/1 -> To Workspace2/1
  From12/1 -> Selector6/1
  Selector6/1 -> To Workspace3/1  "I1"
  [V_dc_pu] -> Gain5/1  "P_mes"
  Gain7/1 -> Sum4/1
  Gain8/1 -> Sum5/2
  Constant1/1 -> Grid_Frame/1(vd_g)
  Constant2/1 -> Grid_Frame/2(vq_g)
  Grid_Frame/2(vabc_0) -> [v_g]
  Demux/1 -> Controlled Voltage Source5/1
  Demux/2 -> Controlled Voltage Source3/1
  Demux/3 -> Controlled Voltage Source4/1
  [v_g] -> Demux/1
  Grid_Frame/1(pho_0) -> Terminator/1
  P_computation/2(Out2) -> [Q_mes]
  From19/1 -> Power/2  "Measured Reactive Power"
  Demux5/2 -> PID Controller5/1  "vq"
  Gain5/1 -> Lead-Lag Filter1/1
  Lead-Lag Filter1/1 -> Sum6/2
  [V_sdq] -> Product2/1
  Ramp/1 -> Sum2/1
  Ramp1/1 -> Sum2/2
  Sum2/1 -> Product2/2
  Demux1/1 -> Transfer Fcn2/1  "vd"
  Demux1/2 -> Gain9/1  "vq"
  Product2/1 -> Demux1/1
  Transfer Fcn1/1 -> Gain11/1
  Transfer Fcn2/1 -> Gain12/1
  Gain11/1 -> Sum5/3
  Gain12/1 -> Sum4/3
  Gain9/1 -> Transfer Fcn1/1
  Sum3/1 -> PID Controller4/1
  P_ref/1 -> Current source calculation and DC Voltage measurement/1(In1)
  Selector4/1 -> To Workspace/1  "Measured Active Power"
  connections:
  Three-Phase Series RLC Branch/LConn1 -- Three-Phase V-I Measurement1/RConn1
  Three-Phase Series RLC Branch/LConn2 -- Three-Phase V-I Measurement1/RConn2
  Three-Phase Series RLC Branch/LConn3 -- Three-Phase V-I Measurement1/RConn3
  Three-Phase V-I Measurement2/LConn1 -- Three-Phase Series RLC Branch/RConn1 -- Three-Phase Series RLC Branch1/LConn1
  Three-Phase V-I Measurement2/LConn2 -- Three-Phase Series RLC Branch/RConn2 -- Three-Phase Series RLC Branch1/LConn2
  Three-Phase Series RLC Branch/RConn3 -- Three-Phase V-I Measurement2/LConn3 -- Three-Phase Series RLC Branch1/LConn3
  Ground/LConn1 -- Three-Phase Series RLC Branch1/RConn3 -- Three-Phase Series RLC Branch1/RConn1 -- Three-Phase Series RLC Branch1/RConn2
  Controlled Voltage Source/RConn1 -- Three-Phase V-I Measurement1/LConn1
  Controlled Voltage Source1/RConn1 -- Three-Phase V-I Measurement1/LConn2
  Controlled Voltage Source2/RConn1 -- Three-Phase V-I Measurement1/LConn3
  Controlled Voltage Source2/LConn1 -- Controlled Voltage Source1/LConn1 -- Controlled Voltage Source/LConn1
  Three-Phase V-I Measurement2/RConn1 -- Three-Phase V-I Measurement7/RConn1 -- SIaD Tool/RConn1
  Three-Phase V-I Measurement2/RConn2 -- Three-Phase V-I Measurement7/RConn2 -- SIaD Tool/RConn2
  Three-Phase V-I Measurement2/RConn3 -- SIaD Tool/RConn3 -- Three-Phase V-I Measurement7/RConn3
  Three-Phase V-I Measurement7/LConn1 -- Three-Phase Series RLC Branch2/LConn1 -- SIaD Tool/LConn1
  Three-Phase V-I Measurement7/LConn2 -- Three-Phase Series RLC Branch2/LConn2 -- SIaD Tool/LConn2
  Three-Phase V-I Measurement7/LConn3 -- Three-Phase Series RLC Branch2/LConn3 -- SIaD Tool/LConn3
  Parallel RLC Branch/RConn1 -- Controlled Current Source/LConn1 -- Controlled Current Source1/RConn1 -- Voltage Measurement/LConn2
  Voltage Measurement/LConn1 -- Controlled Current Source/RConn1 -- Parallel RLC Branch/LConn1 -- Controlled Current Source1/LConn1
  Controlled Voltage Source5/LConn1 -- Controlled Voltage Source4/LConn1 -- Controlled Voltage Source3/LConn1
  Controlled Voltage Source5/RConn1 -- Three-Phase Series RLC Branch2/RConn1
  Controlled Voltage Source3/RConn1 -- Three-Phase Series RLC Branch2/RConn2
  Controlled Voltage Source4/RConn1 -- Three-Phase Series RLC Branch2/RConn3

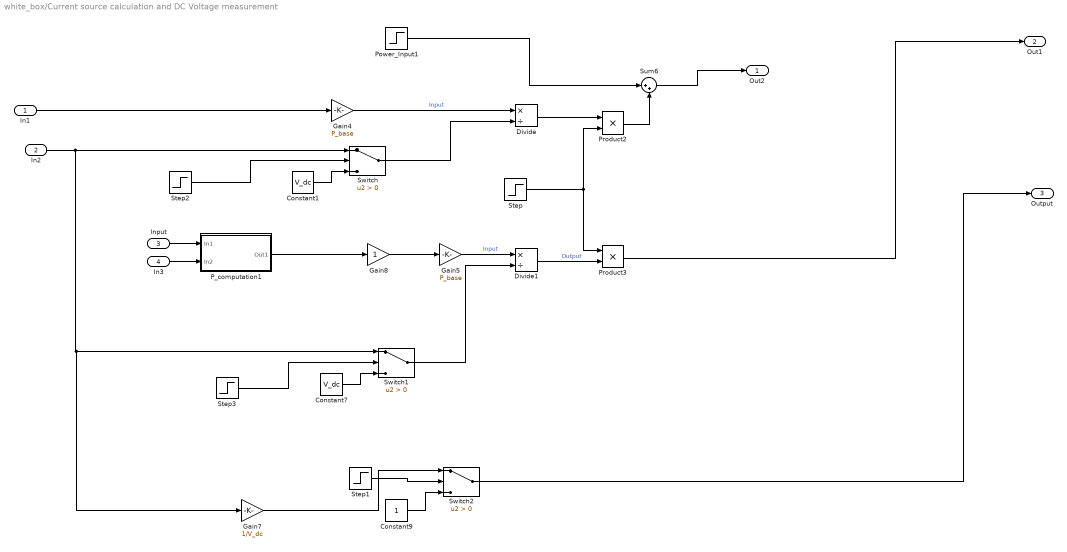
== system white_box/Current source calculation and DC Voltage measurement ==
  In1 : Inport
  In2 : Inport  Port=2
  Input : Inport  Port=3
  In3 : Inport  Port=4
  Constant1 : Constant  Value=V_dc
  Constant7 : Constant  Value=V_dc
  Constant9 : Constant
  Divide : Product  Inputs=*/
  Divide1 : Product  Inputs=*/
  Gain4 : Gain  Gain=P_base
  Gain5 : Gain  Gain=P_base
  Gain7 : Gain  Gain=1/V_dc
  Gain8 : Gain
  P_computation1 : Subsystem
  Power_Input1 : Step  Time=t_charge  Before=I_charge  After=0  SampleTime=0
  Product2 : Product
  Product3 : Product
  Step : Step  Time=t_charge + 0.1  SampleTime=0
  Step1 : Step  Time=0.6  SampleTime=0
  Step2 : Step  Time=0.1  SampleTime=0
  Step3 : Step  Time=0.1  SampleTime=0
  Sum6 : Sum  Inputs=|++
  Switch : Switch  Criteria=u2 > Threshold  SaturateOnIntegerOverflow=off  InputSameDT=off
  Switch1 : Switch  Criteria=u2 > Threshold  SaturateOnIntegerOverflow=off  InputSameDT=off
  Switch2 : Switch  Criteria=u2 > Threshold  SaturateOnIntegerOverflow=off  InputSameDT=off
  Out2 : Outport
  Out1 : Outport  Port=2
  Output : Outport  Port=3
  wires:
  Step3/1 -> Switch1/2
  In1/1 -> Gain4/1
  Constant1/1 -> Switch/3
  Product3/1 -> Out1/1
  Step/1 -> Product3/1, Product2/2
  Divide/1 -> Product2/1
  Gain8/1 -> Gain5/1
  Constant7/1 -> Switch1/3
  Divide1/1 -> Product3/2  "Output"
  Product2/1 -> Sum6/2
  Gain5/1 -> Divide1/1  "Input"
  Power_Input1/1 -> Sum6/1
  Step2/1 -> Switch/2
  P_computation1/1(Out1) -> Gain8/1
  Switch/1 -> Divide/2
  Gain4/1 -> Divide/1  "Input"
  Switch1/1 -> Divide1/2
  Sum6/1 -> Out2/1
  Input/1 -> P_computation1/1(In1)
  In3/1 -> P_computation1/2(In2)
  Step1/1 -> Switch2/2
  Switch2/1 -> Output/1
  Gain7/1 -> Switch2/1
  In2/1 -> Gain7/1, Switch1/1, Switch/1
  Constant9/1 -> Switch2/3

== system white_box/Grid_Frame ==
  vd_g : Inport
  vq_g : Inport  Port=2
  Angle Step : Step  Time=100  After=0.4712  SampleTime=0
  Constant1 : Constant  Value=omega_b
  Gain7 : Gain  Gain=V_base/sqrt(3) * sqrt(2)
  Integrator with Wrapped State (Discrete or Continuous)2 : eeGeneralControl/Integrator with Wrapped State (Discrete or Continuous)  LabelModeActiveChoice=Discrete  WrappedStateUpperValue=2*pi  WrappedStateLowerValue=0  x0=0  Ts=-1
  Mux1 : Mux  Inputs=3
  Product : Product
  Sum : Sum  Inputs=+|+
  Voltage Step : Step  Time=100  Before=1  After=0.95  SampleTime=0
  dq0 to abc1 : spsdq0toabcLib/dq0 to abc  Alignment=90 degrees behind phase A axis
  pho_0 : Outport
  vabc_0 : Outport  Port=2
  wires:
  Constant1/1 -> Integrator with Wrapped State (Discrete or Continuous)2/1
  Mux1/1 -> dq0 to abc1/1
  dq0 to abc1/1 -> Gain7/1  "vabc_ef"
  Gain7/1 -> Product/1
  vd_g/1 -> Mux1/1  "vd_g"
  vq_g/1 -> Mux1/3, Mux1/2  "vq_g"
  Angle Step/1 -> Sum/1
  Integrator with Wrapped State (Discrete or Continuous)2/1 -> Sum/2  "pho_0"
  Sum/1 -> pho_0/1, dq0 to abc1/2
  Product/1 -> vabc_0/1
  Voltage Step/1 -> Product/2

== system white_box/P_computation ==
  In1 : Inport
  In2 : Inport  Port=2
  Demux2 : Demux  Outputs=2
  Demux3 : Demux  Outputs=2
  Product{,1..3} (4 alike) : Product
  Sum : Sum  Inputs=|++
  Sum1 : Sum  Inputs=|+-
  Out1 : Outport
  Out2 : Outport  Port=2
  wires:
  In1/1 -> Demux2/1
  In2/1 -> Demux3/1
  Demux2/2 -> Product1/1
  Product/1 -> Sum/1
  Product1/1 -> Sum/2
  Sum/1 -> Out1/1
  Product3/1 -> Sum1/2
  Demux3/1 -> Product2/2, Product2/1, Product/2
  Product2/1 -> Sum1/1
  Demux3/2 -> Product3/2, Product1/2
  Demux2/1 -> Product3/1, Product/1
  Sum1/1 -> Out2/1

== system white_box/SIaD Tool ==
  Decoupled State : Subsystem
      settings: PortSchema="{\"entries\":[{\"content\":{\"sides\":[{\"content\":{\"connectorIds\":[\"LConn1\",\"LConn2\",\"LConn3\"]},\"type\":\"ConnectorPlacement.EquallySpacedRectSide\",\"uuid\":\"d0026cad-bf69-43aa-99db-8cc8562f1524\"},{\"content\":{\"side\":\"RIGHT\"},\"type\":\"ConnectorPlacement.EquallySpacedRectSide\",\"uuid\":\"64b8bea8-dfd1-490d-8772-f15621dca227\"},{\"content\":{\"connectorIds\":[\"LConn4\",\"LConn5\",\"LConn6\"],\"side\":\"TOP\"},\"type\":\"ConnectorPlacement.EquallySpacedRectSide\",\"uuid\":\"5c20e442-7542-4d44-8051-809eca545f48\"},{\"content\":{\"connectorIds\":[\"RConn1\",\"RConn2\",\"RConn3\"],\"side\":\"BOTTOM\"},\"type\":\"ConnectorPlacement.EquallySpacedRectSide\",\"uuid\":\"0dac49be-ef95-43f1-976a-782473b2e343\"}]},\"type\":\"ConnectorPlacement.EquallySpacedConnector\",\"uuid\":\"aff4678d-8b0f-4c58-9998-b2e98e043de0\"}],\"packageUris\":[\"http://schema.mathworks.com/mf0/Connector/R2020b\"],\"version\":\"1.0\"}"
  Frequency Scanner : Subsystem  Commented=on
  Normal State : Subsystem
  Steady State : Subsystem
  System 1 : Subsystem  Commented=on
  System 1 Meas : spsThreePhaseVIMeasurementLib/Three-Phase V-I Measurement  VoltageMeasurement=phase-to-ground  SetLabelV=on  LabelV=Vabc1  Vpu=off  VpuLL=off  CurrentMeasurement=yes  SetLabelI=on  LabelI=Iabc1  Ipu=off  Pbase=100e6  Vbase=500e3  OutputType=Complex  PhasorSimulation=off  PSBequivalent=0
  System 2 : Subsystem  Commented=on
  System 2 Meas : spsThreePhaseVIMeasurementLib/Three-Phase V-I Measurement  VoltageMeasurement=phase-to-ground  SetLabelV=on  LabelV=Vabc2  Vpu=off  VpuLL=off  CurrentMeasurement=yes  SetLabelI=on  LabelI=Iabc2  Ipu=off  Pbase=100e6  Vbase=500e3  OutputType=Complex  PhasorSimulation=off  PSBequivalent=0
  A2 : PMIOPort  Side=Left
  B2 : PMIOPort  Port=2  Side=Left
  C2 : PMIOPort  Port=3  Side=Left
  A1 : PMIOPort  Port=4  Side=Right
  B1 : PMIOPort  Port=5  Side=Right
  C1 : PMIOPort  Port=6  Side=Right
  wires:
  [Vabc1] -> Steady State/1(Voltage)
  [Iabc1] -> Steady State/2(Current)
  [Iabc1] -> System 1/2(Current1)
  [Vabc1] -> System 1/1(Voltage1)
  [Vabc2] -> System 2/1(Voltage2)
  [Iabc2] -> System 2/2(Current2)
  connections:
  Normal State/LConn1 -- System 1 Meas/LConn1 -- Decoupled State/LConn6
  Normal State/RConn3 -- System 2 Meas/LConn3 -- Decoupled State/RConn1
  Decoupled State/LConn5 -- System 1 Meas/LConn2 -- Normal State/LConn2
  Normal State/LConn3 -- System 1 Meas/LConn3 -- Decoupled State/LConn4
  Normal State/RConn1 -- System 2 Meas/LConn1 -- Decoupled State/RConn3
  Normal State/RConn2 -- System 2 Meas/LConn2 -- Decoupled State/RConn2
  Decoupled State/LConn1 -- Frequency Scanner/LConn1
  Decoupled State/LConn2 -- Frequency Scanner/LConn2
  Decoupled State/LConn3 -- Frequency Scanner/LConn3
  System 1 Meas/RConn1 -- A1/RConn1
  System 1 Meas/RConn2 -- B1/RConn1
  System 1 Meas/RConn3 -- C1/RConn1
  System 2 Meas/RConn1 -- A2/RConn1
  System 2 Meas/RConn2 -- B2/RConn1
  System 2 Meas/RConn3 -- C2/RConn1

== system white_box/Vpoc_computation ==
  In1 : Inport
  Demux2 : Demux  Outputs=2
  Sqrt : Sqrt
  Square : Math  Operator=square
  Square1 : Math  Operator=square
  Sum6 : Sum  Inputs=|++
  Out1 : Outport
  wires:
  Sqrt/1 -> Out1/1
  Sum6/1 -> Sqrt/1
  Demux2/1 -> Square/1
  Square1/1 -> Sum6/2
  In1/1 -> Demux2/1
  Square/1 -> Sum6/1
  Demux2/2 -> Square1/1

== system white_box/Current source calculation and DC Voltage measurement/P_computation1 ==
  In1 : Inport
  In2 : Inport  Port=2
  Demux2 : Demux  Outputs=2
  Demux3 : Demux  Outputs=2
  Product : Product
  Product1 : Product
  Sum : Sum  Inputs=|++
  Out1 : Outport
  wires:
  In1/1 -> Demux2/1
  In2/1 -> Demux3/1
  Demux2/1 -> Product/1
  Demux3/1 -> Product/2
  Demux2/2 -> Product1/1
  Demux3/2 -> Product1/2
  Product/1 -> Sum/1
  Product1/1 -> Sum/2
  Sum/1 -> Out1/1

== system white_box/SIaD Tool/Decoupled State ==
  Three-Phase V-I Measurement7 : spsThreePhaseVIMeasurementLib/Three-Phase V-I Measurement  VoltageMeasurement=no  SetLabelV=on  LabelV=Vabc  Vpu=off  VpuLL=off  CurrentMeasurement=no  SetLabelI=on  LabelI=Iabc  Ipu=off  Pbase=100e6  Vbase=500e3  OutputType=Complex  PhasorSimulation=off  PSBequivalent=0
  Three-Phase V-I Measurement8 : spsThreePhaseVIMeasurementLib/Three-Phase V-I Measurement  VoltageMeasurement=no  SetLabelV=on  LabelV=Vabc  Vpu=off  VpuLL=off  CurrentMeasurement=no  SetLabelI=on  LabelI=Iabc  Ipu=off  Pbase=100e6  Vbase=500e3  OutputType=Complex  PhasorSimulation=off  PSBequivalent=0
  A : PMIOPort  Side=Left
  B : PMIOPort  Port=2  Side=Left
  C : PMIOPort  Port=3  Side=Left
  S1c : PMIOPort  Port=4  Side=Left
  S1b : PMIOPort  Port=5  Side=Left
  S1a : PMIOPort  Port=6  Side=Left
  S2c : PMIOPort  Port=7  Side=Right
  S2b : PMIOPort  Port=8  Side=Right
  S2a : PMIOPort  Port=9  Side=Right
  connections:
  S1a/RConn1 -- S2a/RConn1 -- Three-Phase V-I Measurement7/LConn1
  A/RConn1 -- Three-Phase V-I Measurement8/RConn1
  B/RConn1 -- Three-Phase V-I Measurement8/RConn2
  C/RConn1 -- Three-Phase V-I Measurement8/RConn3
  Three-Phase V-I Measurement8/LConn1 -- Three-Phase V-I Measurement7/RConn1
  Three-Phase V-I Measurement8/LConn2 -- Three-Phase V-I Measurement7/RConn2
  Three-Phase V-I Measurement8/LConn3 -- Three-Phase V-I Measurement7/RConn3
  S1b/RConn1 -- S2b/RConn1 -- Three-Phase V-I Measurement7/LConn2
  S1c/RConn1 -- S2c/RConn1 -- Three-Phase V-I Measurement7/LConn3

== system white_box/SIaD Tool/Frequency Scanner ==
  note: Current perturbation method
  note: Voltage perturbation method
  Current Strategy : Subsystem  Commented=on
  Three-Phase V-I Measurement1 : spsThreePhaseVIMeasurementLib/Three-Phase V-I Measurement  VoltageMeasurement=no  SetLabelV=on  LabelV=Vabc  Vpu=off  VpuLL=off  CurrentMeasurement=no  SetLabelI=on  LabelI=Iabc  Ipu=off  Pbase=100e6  Vbase=500e3  OutputType=Complex  PhasorSimulation=off  PSBequivalent=0
  Three-Phase V-I Measurement3 : spsThreePhaseVIMeasurementLib/Three-Phase V-I Measurement  VoltageMeasurement=no  SetLabelV=on  LabelV=Vabc  Vpu=off  VpuLL=off  CurrentMeasurement=no  SetLabelI=on  LabelI=Iabc  Ipu=off  Pbase=100e6  Vbase=500e3  OutputType=Complex  PhasorSimulation=off  PSBequivalent=0
  Voltage Strategy : Subsystem
  a : PMIOPort  Side=Left
  b : PMIOPort  Port=2  Side=Left
  c : PMIOPort  Port=3  Side=Left
  connections:
  Three-Phase V-I Measurement3/LConn2 -- Current Strategy/LConn2
  Three-Phase V-I Measurement3/RConn3 -- Three-Phase V-I Measurement1/RConn3 -- c/RConn1
  Three-Phase V-I Measurement3/RConn1 -- a/RConn1 -- Three-Phase V-I Measurement1/RConn1
  Three-Phase V-I Measurement3/LConn1 -- Current Strategy/LConn1
  Three-Phase V-I Measurement3/RConn2 -- Three-Phase V-I Measurement1/RConn2 -- b/RConn1
  Three-Phase V-I Measurement3/LConn3 -- Current Strategy/LConn3
  Three-Phase V-I Measurement1/LConn1 -- Voltage Strategy/RConn1
  Three-Phase V-I Measurement1/LConn3 -- Voltage Strategy/RConn3
  Three-Phase V-I Measurement1/LConn2 -- Voltage Strategy/RConn2

== system white_box/SIaD Tool/Normal State ==
  Three-Phase V-I Measurement7 : spsThreePhaseVIMeasurementLib/Three-Phase V-I Measurement  VoltageMeasurement=no  SetLabelV=on  LabelV=Vabc  Vpu=off  VpuLL=off  CurrentMeasurement=no  SetLabelI=on  LabelI=Iabc  Ipu=off  Pbase=100e6  Vbase=500e3  OutputType=Complex  PhasorSimulation=off  PSBequivalent=0
  Three-Phase V-I Measurement8 : spsThreePhaseVIMeasurementLib/Three-Phase V-I Measurement  VoltageMeasurement=no  SetLabelV=on  LabelV=Vabc  Vpu=off  VpuLL=off  CurrentMeasurement=no  SetLabelI=on  LabelI=Iabc  Ipu=off  Pbase=100e6  Vbase=500e3  OutputType=Complex  PhasorSimulation=off  PSBequivalent=0
  a : PMIOPort  Side=Right
  A : PMIOPort  Port=2  Side=Left
  b : PMIOPort  Port=3  Side=Right
  B : PMIOPort  Port=4  Side=Left
  c : PMIOPort  Port=5  Side=Right
  C : PMIOPort  Port=6  Side=Left
  connections:
  Three-Phase V-I Measurement7/LConn2 -- Three-Phase V-I Measurement8/RConn2
  Three-Phase V-I Measurement7/RConn2 -- b/RConn1
  Three-Phase V-I Measurement7/LConn3 -- Three-Phase V-I Measurement8/RConn3
  Three-Phase V-I Measurement7/LConn1 -- Three-Phase V-I Measurement8/RConn1
  Three-Phase V-I Measurement7/RConn3 -- c/RConn1
  Three-Phase V-I Measurement8/LConn1 -- A/RConn1
  Three-Phase V-I Measurement8/LConn3 -- C/RConn1
  Three-Phase V-I Measurement7/RConn1 -- a/RConn1
  Three-Phase V-I Measurement8/LConn2 -- B/RConn1

== system white_box/SIaD Tool/Steady State ==
  note: Voltage measurements
  note: Voltage measurements
  Voltage : Inport
  Current : Inport  Port=2
  Demux1 : Demux  Outputs=3
  Demux2 : Demux  Outputs=3
  Fortescue Transformation : Subsystem
  Fortescue Transformation1 : Subsystem
  Mux1 : Mux  Inputs=2
  Mux2 : Mux  Inputs=2
  PLL (3ph) : spsPLL3phLib/PLL (3ph)  Fmin=45  Par_Init=[0, f0]  ParK=[180, 3200, 1]  TcD=1e-4  MaxRateChangeFreq=12  FilterCutOffFreq=25  Ts=delta_t  AGC=on
  Park Transform1 : Subsystem
  Park Transform2 : Subsystem
  Terminator1 : Terminator
  Terminator2 : Terminator
  Terminator4 : Terminator
  To Workspace1 : ToWorkspace  VariableName=Vabc_ss  SampleTime=-1
  To Workspace2 : ToWorkspace  VariableName=Iabc_ss  SampleTime=-1
  To Workspace22 : ToWorkspace  VariableName=Vdq_ss  SampleTime=-1
  To Workspace3 : ToWorkspace  VariableName=Idq_ss  SampleTime=-1
  To Workspace4 : ToWorkspace  VariableName=I0pn_ss  SampleTime=-1
  To Workspace7 : ToWorkspace  VariableName=V0pn_ss  SampleTime=-1
  wires:
  Demux2/3 -> Terminator2/1
  PLL (3ph)/2 -> [wt_ss], Park Transform2/2(wt)
  Voltage/1 -> Fortescue Transformation/1(ABC), PLL (3ph)/1, Park Transform2/1(ABC), To Workspace1/1
  PLL (3ph)/1 -> Terminator1/1
  Mux2/1 -> To Workspace22/1
  Fortescue Transformation/1(0PN) -> To Workspace7/1
  Demux2/1 -> Mux2/1
  Park Transform2/1(qd0) -> Demux2/1
  Demux2/2 -> Mux2/2
  Park Transform1/1(qd0) -> Demux1/1
  Demux1/1 -> Mux1/1
  Fortescue Transformation1/1(0PN) -> To Workspace4/1
  Mux1/1 -> To Workspace3/1
  Demux1/3 -> Terminator4/1
  Current/1 -> Fortescue Transformation1/1(ABC), To Workspace2/1, Park Transform1/1(ABC)
  Demux1/2 -> Mux1/2
  [wt_ss] -> Park Transform1/2(wt)

== system white_box/SIaD Tool/System 1 ==
  Voltage1 : Inport
  Current1 : Inport  Port=2
  0pn Sequence : Subsystem  Commented=on
  ABC Sequence : Subsystem  Commented=on
  dq0 Sequence : Subsystem
  wires:
  Voltage1/1 -> 0pn Sequence/1(Vabc), dq0 Sequence/1(Vabc), ABC Sequence/1(Vabc)
  Current1/1 -> 0pn Sequence/2(Iabc), dq0 Sequence/2(Iabc), ABC Sequence/2(Iabc)

== system white_box/SIaD Tool/System 2 ==
  Voltage2 : Inport
  Current2 : Inport  Port=2
  0pn Sequence : Subsystem  Commented=on
  ABC Sequence : Subsystem  Commented=on
  dq0 Sequence : Subsystem
  wires:
  Voltage2/1 -> 0pn Sequence/1(Vabc), dq0 Sequence/1(Vabc), ABC Sequence/1(Vabc)
  Current2/1 -> 0pn Sequence/2(Iabc), dq0 Sequence/2(Iabc), ABC Sequence/2(Iabc)
